simulink model "Modello_Lineare"  (R2025b)
settings: Solver=VariableStepAuto  StartTime=0.0  StopTime=500  RelTol=1e-3
values from neighbouring files (symbols this model uses):
  C = [1, 0, 0]    [fase1.m]
  yeq = xeq(1,:)    [fase1.m]
undefined symbols (not defined in the file or in its folder): A, B, D, ueq
settings Model: Creator=Rika  LastModifiedBy=Rika

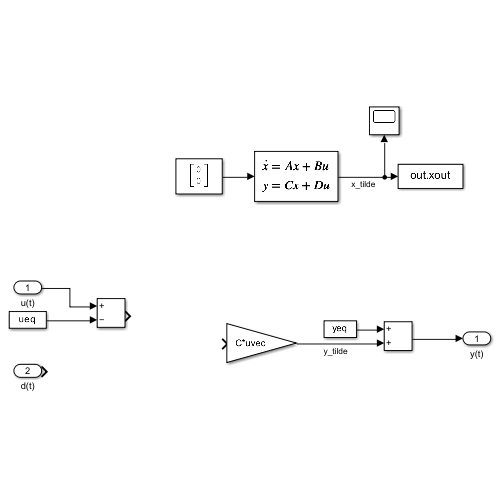
[thumbnail: Simulink's stored preview of the top-level diagram]
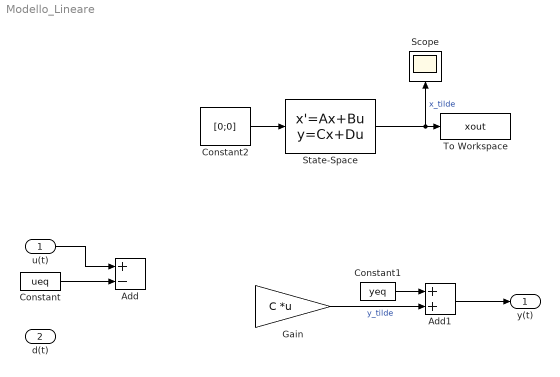
== system Modello_Lineare ==
  u(t) : Inport
  d(t) : Inport  Port=2
  Add : Sum  Inputs=+-
  Add1 : Sum
  Constant : Constant  Value=ueq
  Constant1 : Constant  Value=yeq
  Constant2 : Constant  Value=[0;0]  VectorParams1D=off
  Gain : Gain  Gain=C  Multiplication=Matrix(K*u) (u vector)
  Scope : Scope
      settings: ActiveDisplayYMinimum=-1  ActiveDisplayYMaximum=1
  State-Space : StateSpace  A=A  B=B  C=C  D=D  InitialCondition=[50;0;20]
  To Workspace : ToWorkspace  VariableName=xout  SaveFormat=Timeseries  SampleTime=-1
  y(t) : Outport
  wires:
  Gain/1 -> Add1/2  "y_tilde"
  State-Space/1 -> Scope/1, To Workspace/1  "x_tilde"
  Constant1/1 -> Add1/1
  Constant/1 -> Add/2
  u(t)/1 -> Add/1
  Add1/1 -> y(t)/1
  Constant2/1 -> State-Space/1
